simulink model "F16ASYM_Controlled"  (R2015a)
settings: Solver=ode3  SolverMode=SingleTasking  StartTime=0.0  StopTime=inf  FixedStep=T_sim  RelTol=1e-3
InitFcn:
  | load('NN_c_weights_Last_stable.mat')
StopFcn:
  | Final_results
values from neighbouring files (symbols this model uses):
  a1 = fitresult.p1    [Stall_protection.m]
  alpha_map_eval = ones(size(M_eval))*NaN    [Auto_trim_aid.m]    (also in Autotrim_maps.mat = [nan nan 0.277598136245 0.119432432992 0.0579479097061 0.027)
  beta_map_eval = ones(size(M_eval))*NaN    [Auto_trim_aid.m]    (also in Autotrim_maps.mat = [nan nan -0.00151549403324 0.00117807579006 -0.0052086799721)
  C_L_0 = fitresult.p2    [Stall_protection.m]
  G_eval = NaN*ones(size(M_sq,2),size(H_sq,2))    [Stall_protection.m]
  H_sq = unique(sort(H_sq))    [Stall_protection.m]
  H_sq_autotrim = min( F_envelope.H_1g):2000:max(F_envelope.H_1g)    [Auto_trim_aid.m]    (also in Autotrim_maps.mat = [0 2000 4000 6000 8000 10000 12000 14000 16000 18000])
  K_b_q_extrap_ACC = K_b_q_extrap    [RUN_ME.m]
  K_b_q_extrap_AoA = K_b_q_extrap    [RUN_ME.m]
  M_sq = unique(sort(M_sq))    [Stall_protection.m]
  M_sq_autotrim = 0:0.1:max(F_envelope.M_1g)    [Auto_trim_aid.m]    (also in Autotrim_maps.mat = [0 0.1 0.2 0.3 0.4 0.5 0.6 0.7 0.8 0.9 1 1.1 ... (21 element)
  T_sim = 0.02    [RUN_ME.m]
  tau_q_extrap_ACC = tau_q_extrap    [RUN_ME.m]
  tau_q_extrap_AoA = tau_q_extrap    [RUN_ME.m]
  velocity = M_eval(I,J)*a    [Auto_trim_aid.m]
undefined symbols (not defined in the file or in its folder): ACCEL, B, Earth, fi_flag_Simulink, GYRO, H_sq_sche, k_B, K_b_ACC_extrap, K_b_AoA_extrap, latitude, longitude, m, m_B, M_sq_sche, Model_used_flag, rad, s, sigbuilder_block, Stall_curve, tau_ACC_extrap, tau_AoA_extrap, Theta_1_roll_last, Theta_2_roll_last, Theta_3_roll_last, trim_control, trim_state, trim_throttle, V_Comp_A_w_z_last, V_Comp_last, V_Comp_last_ONE, V_long_lastA_w_z, V_long_lastAoA, V_roll_last, V_roll_lastMOD, V_yaw_last, W_Comp_A_w_z_last, W_Comp_last, W_long_lastA_w_z, W_long_lastAoA, W_roll_last, W_roll_lastMOD, W_yaw_last, WGS84
libraries: Adaptive_FaultTolerantControl x57, dspsigops x37, F16_Actuator_Library x14, commnoisgen2 x13, simulink x11, simulink_extras x10, dsparch4 x6, aerolibatmos2 x6, aerolibtransform2 x6, aerolibfltsims x3, dspvision x3, dspsnks4 x3
(part 11 of 14)

== system F16ASYM_Controlled/Primary Controller/P con  + Crossed NN + AWU+Lim + hand-over+Scheduling/P controller + adaptive Crossed NN + AWU+Lim   in AoA/Physical limitation/Moments ==
  C_L : Inport
  C_M : Inport  Port=2
  C_N : Inport  Port=3
  q : Inport  Port=4
  B span : Constant  Value=9.144
  CMA : Constant  Value=3.45
  Divide : Product  Inputs=**
  Divide1 : Product  Inputs=***
  Divide2 : Product  Inputs=**
  Divide3 : Product  Inputs=***
  Divide4 : Product  Inputs=**
  S_w : Constant  Value=27.87
  S_w1 : Constant  Value=27.87
  q1 : InportShadow  Port=4
  L : Outport
  M : Outport  Port=2
  N : Outport  Port=3
  wires:
  q/1 -> Divide1/1
  S_w/1 -> Divide1/2
  B span/1 -> Divide1/3
  C_L/1 -> Divide/1
  Divide1/1 -> Divide2/1, Divide/2
  Divide/1 -> L/1  "L"
  C_N/1 -> Divide2/2
  Divide2/1 -> N/1  "N"
  q1/1 -> Divide3/1
  S_w1/1 -> Divide3/2
  CMA/1 -> Divide3/3
  C_M/1 -> Divide4/1
  Divide3/1 -> Divide4/2
  Divide4/1 -> M/1  "M"

== system F16ASYM_Controlled/Primary Controller/P con + Crossed NN + AWU+Lim + hand-over/P controller + adaptive Crossed NN + AWU+Lim    in ACC /Long Dyn Inversion: alpha_dot ->q/Completed ==
  alpha_dot_c : Inport
  All_meas : Inport  Port=2
  A_w_z : Selector  InputPortWidth=3  Indices=3
  Add : Sum
  Bus Selector : BusSelector  OutputSignals=signal1.AoA meas (rad),signal1.omega_b meas (rad/s),signal1.SS meas (rad),signal1.V_TAS (m/s),signal2.A_w_CG
  Display : Display
  Display1 : Display
  Display2 : Display
  Divide{,1..3} (4 alike) : Product  Inputs=**
  Divide4 : Product  Inputs=/*
  Selector : Selector  InputPortWidth=3
  Selector1 : Selector  InputPortWidth=3  Indices=3
  Trigonometric Function : Trigonometry  Operator=sincos
  Trigonometric Function1 : Trigonometry  Operator=tan
  Trigonometric Function2 : Trigonometry  Operator=cos
  "q_c " : Sum  Inputs=++-
  q_c : Outport
  wires:
  Trigonometric Function/1 -> Divide1/1
  Bus Selector/1 -> Trigonometric Function/1  "<AoA meas (rad)>"
  Selector/1 -> Divide/2
  Bus Selector/2 -> Selector1/1, Selector/1  "<omega_b meas (rad/s)>"
  Divide2/1 -> "q_c "/2, Display1/1
  Selector1/1 -> Divide1/2
  Divide3/1 -> Divide4/1
  alpha_dot_c/1 -> "q_c "/1, Display/1
  All_meas/1 -> Bus Selector/1
  Bus Selector/5 -> A_w_z/1  "<A_w_CG>"
  Bus Selector/3 -> Trigonometric Function1/1, Trigonometric Function2/1  "<SS meas (rad)>"
  Divide4/1 -> "q_c "/3
  "q_c "/1 -> q_c/1
  Divide/1 -> Add/1
  Bus Selector/4 -> Divide3/2  "<V_TAS (m/s)>"
  Add/1 -> Divide2/1
  Trigonometric Function1/1 -> Divide2/2
  Divide1/1 -> Add/2
  Trigonometric Function2/1 -> Divide3/1
  Trigonometric Function/2 -> Divide/1
  A_w_z/1 -> Display2/1, Divide4/2

== system F16ASYM_Controlled/Primary Controller/P con + Crossed NN + AWU+Lim + hand-over/P controller + adaptive Crossed NN + AWU+Lim    in ACC /Long Dyn Inversion: alpha_dot ->q/Simplified ==
  alpha_dot_c : Inport
  All_meas : Inport  Port=2
  A_b_z : Selector  InputPortWidth=3  Indices=3
  Bus Selector : BusSelector  OutputSignals=signal2.A_b_CG,signal1.V_TAS (m/s)
  Display : Display
  Divide4 : Product  Inputs=*/
  "q_c " : Sum  Inputs=+-
  q_c : Outport
  wires:
  "q_c "/1 -> q_c/1
  All_meas/1 -> Bus Selector/1
  alpha_dot_c/1 -> "q_c "/1, Display/1
  Bus Selector/2 -> Divide4/2  "<V_TAS (m/s)>"
  Divide4/1 -> "q_c "/2
  A_b_z/1 -> Divide4/1  "A_b_z"
  Bus Selector/1 -> A_b_z/1  "<A_b_CG>"

== system F16ASYM_Controlled/Primary Controller/P con + Crossed NN + AWU+Lim + hand-over/P controller + adaptive Crossed NN + AWU+Lim    in ACC /Longitudinal controller in A_w_z/Accel rate --> AoA rate! ==
  All_meas : Inport
  1/a_1 : Gain  Gain=1/a1
  Bus Selector : BusSelector  OutputSignals=signal2.q (Pa)
  Divide : Product  Inputs=**
  Divide2 : Product  Inputs=*/
  S : Constant  Value=27.87
  mass : Constant  Value=9295.44
  A_w  to AoA rates factor : Outport
  wires:
  S/1 -> Divide/1
  Bus Selector/1 -> Divide/2  "<q (Pa)>"
  mass/1 -> Divide2/1
  Divide/1 -> Divide2/2
  Divide2/1 -> 1/a_1/1
  All_meas/1 -> Bus Selector/1
  1/a_1/1 -> A_w  to AoA rates factor/1

== system F16ASYM_Controlled/Primary Controller/P con + Crossed NN + AWU+Lim + hand-over/P controller + adaptive Crossed NN + AWU+Lim    in ACC /Longitudinal controller in A_w_z/Stall protection ==
  alpha_dot des : Inport
  All meas : Inport  Port=2
  Bus Selector : BusSelector  OutputSignals=signal1.AoA meas (rad)
  MATLAB Function : MATLAB Function  TreatAsAtomicUnit=on
  AoA des : Outport
  wires:
  alpha_dot des/1 -> MATLAB Function/1(alpha_dot)
  MATLAB Function/1(alpha_dot_out) -> AoA des/1
  All meas/1 -> Bus Selector/1
  Bus Selector/1 -> MATLAB Function/2(alpha)  "<AoA meas (rad)>"

== system F16ASYM_Controlled/Primary Controller/P con + Crossed NN + AWU+Lim + hand-over/P controller + adaptive Crossed NN + AWU+Lim    in ACC /Physical limitation/Moments ==
  C_L : Inport
  C_M : Inport  Port=2
  C_N : Inport  Port=3
  q : Inport  Port=4
  B span : Constant  Value=9.144
  CMA : Constant  Value=3.45
  Divide : Product  Inputs=**
  Divide1 : Product  Inputs=***
  Divide2 : Product  Inputs=**
  Divide3 : Product  Inputs=***
  Divide4 : Product  Inputs=**
  S_w : Constant  Value=27.87
  S_w1 : Constant  Value=27.87
  q1 : InportShadow  Port=4
  L : Outport
  M : Outport  Port=2
  N : Outport  Port=3
  wires:
  Divide4/1 -> M/1  "M"
  Divide3/1 -> Divide4/2
  C_M/1 -> Divide4/1
  CMA/1 -> Divide3/3
  S_w1/1 -> Divide3/2
  q1/1 -> Divide3/1
  Divide2/1 -> N/1  "N"
  C_N/1 -> Divide2/2
  Divide/1 -> L/1  "L"
  Divide1/1 -> Divide/2, Divide2/1
  C_L/1 -> Divide/1
  B span/1 -> Divide1/3
  S_w/1 -> Divide1/2
  q/1 -> Divide1/1

== system F16ASYM_Controlled/Primary Controller/P con + Crossed NN + AWU+Lim + hand-over/P controller + adaptive Crossed NN + AWU+Lim   in AoA/Long Dyn Inversion: alpha_dot ->q/Completed ==
  alpha_dot_c : Inport
  All_meas : Inport  Port=2
  A_w_z : Selector  InputPortWidth=3  Indices=3
  Add : Sum
  Bus Selector : BusSelector  OutputSignals=signal1.AoA meas (rad),signal1.omega_b meas (rad/s),signal1.SS meas (rad),signal1.V_TAS (m/s),signal2.A_w_CG
  Display : Display
  Display1 : Display
  Display2 : Display
  Divide{,1..3} (4 alike) : Product  Inputs=**
  Divide4 : Product  Inputs=/*
  Selector : Selector  InputPortWidth=3
  Selector1 : Selector  InputPortWidth=3  Indices=3
  Trigonometric Function : Trigonometry  Operator=sincos
  Trigonometric Function1 : Trigonometry  Operator=tan
  Trigonometric Function2 : Trigonometry  Operator=cos
  "q_c " : Sum  Inputs=++-
  q_c : Outport
  wires:
  Trigonometric Function/1 -> Divide1/1
  Bus Selector/1 -> Trigonometric Function/1  "<AoA meas (rad)>"
  Selector/1 -> Divide/2
  Bus Selector/2 -> Selector1/1, Selector/1  "<omega_b meas (rad/s)>"
  Divide2/1 -> "q_c "/2, Display1/1
  Selector1/1 -> Divide1/2
  Divide3/1 -> Divide4/1
  alpha_dot_c/1 -> "q_c "/1, Display/1
  All_meas/1 -> Bus Selector/1
  Bus Selector/5 -> A_w_z/1  "<A_w_CG>"
  Bus Selector/3 -> Trigonometric Function1/1, Trigonometric Function2/1  "<SS meas (rad)>"
  Divide4/1 -> "q_c "/3
  "q_c "/1 -> q_c/1
  Divide/1 -> Add/1
  Bus Selector/4 -> Divide3/2  "<V_TAS (m/s)>"
  Add/1 -> Divide2/1
  Trigonometric Function1/1 -> Divide2/2
  Divide1/1 -> Add/2
  Trigonometric Function2/1 -> Divide3/1
  Trigonometric Function/2 -> Divide/1
  A_w_z/1 -> Display2/1, Divide4/2

== system F16ASYM_Controlled/Primary Controller/P con + Crossed NN + AWU+Lim + hand-over/P controller + adaptive Crossed NN + AWU+Lim   in AoA/Long Dyn Inversion: alpha_dot ->q/Simplified ==
  alpha_dot_c : Inport
  All_meas : Inport  Port=2
  A_b_z : Selector  InputPortWidth=3  Indices=3
  Bus Selector : BusSelector  OutputSignals=signal2.A_b_CG,signal1.V_TAS (m/s)
  Display : Display
  Divide4 : Product  Inputs=*/
  "q_c " : Sum  Inputs=+-
  q_c : Outport
  wires:
  "q_c "/1 -> q_c/1
  All_meas/1 -> Bus Selector/1
  alpha_dot_c/1 -> "q_c "/1, Display/1
  Bus Selector/2 -> Divide4/2  "<V_TAS (m/s)>"
  Divide4/1 -> "q_c "/2
  A_b_z/1 -> Divide4/1  "A_b_z"
  Bus Selector/1 -> A_b_z/1  "<A_b_CG>"

== system F16ASYM_Controlled/Primary Controller/P con + Crossed NN + AWU+Lim + hand-over/P controller + adaptive Crossed NN + AWU+Lim   in AoA/Physical limitation/Moments ==
  C_L : Inport
  C_M : Inport  Port=2
  C_N : Inport  Port=3
  q : Inport  Port=4
  B span : Constant  Value=9.144
  CMA : Constant  Value=3.45
  Divide : Product  Inputs=**
  Divide1 : Product  Inputs=***
  Divide2 : Product  Inputs=**
  Divide3 : Product  Inputs=***
  Divide4 : Product  Inputs=**
  S_w : Constant  Value=27.87
  S_w1 : Constant  Value=27.87
  q1 : InportShadow  Port=4
  L : Outport
  M : Outport  Port=2
  N : Outport  Port=3
  wires:
  Divide4/1 -> M/1  "M"
  Divide3/1 -> Divide4/2
  C_M/1 -> Divide4/1
  CMA/1 -> Divide3/3
  S_w1/1 -> Divide3/2
  q1/1 -> Divide3/1
  Divide2/1 -> N/1  "N"
  C_N/1 -> Divide2/2
  Divide/1 -> L/1  "L"
  Divide1/1 -> Divide/2, Divide2/1
  C_L/1 -> Divide/1
  B span/1 -> Divide1/3
  S_w/1 -> Divide1/2
  q/1 -> Divide1/1

== system F16ASYM_Controlled/Primary Controller/P con + adaptive Crossed NN + AWU+Lim + Scheduling/Body Rates Controller/Body Rates Controller  in ACC/Ref Model and P Controller1 ==
  y_ref : Inport
  y_meas : Inport  Port=2
  All meas : Inport  Port=3
  " " : Sum  Inputs=|+-
  2-D Lookup Table1 : Lookup_n-D  BreakpointsForDimension1=M_sq_sche  BreakpointsForDimension2=H_sq_sche  BeginIndexSearchUsingPreviousIndexResult=on  Table=tau_q_extrap_ACC  ExtrapMethod=Clip  RemoveProtectionInput=on  UseLastTableValue=on  SampleTime=2*T_sim  RndMeth=Simplest  InputSameDT=on
  2-D Lookup Table2 : Lookup_n-D  BreakpointsForDimension1=M_sq_sche  BreakpointsForDimension2=H_sq_sche  BeginIndexSearchUsingPreviousIndexResult=on  Table=K_b_q_extrap_ACC  ExtrapMethod=Clip  RemoveProtectionInput=on  UseLastTableValue=on  SampleTime=2*T_sim  RndMeth=Simplest  InputSameDT=on
  Add1 : Sum  Inputs=++|
  Bus Selector1 : BusSelector  OutputSignals=signal2.Mach,signal1.Alt meas (m)
  Divide : Product  Inputs=**
  K_f : Gain
  Reference Model : Subsystem
  Saturation : Saturate  UpperLimit=1  LowerLimit=2*T_sim
  Saturation1 : Saturate  UpperLimit=10  LowerLimit=0.1
  Switch1 : Switch  Threshold=0.5
  Switch2 : Switch  Threshold=0.5
  def : Constant
  isNaN1 : RelationalOperator  Operator=isNaN  OutDataTypeStr=boolean
  isNaN2 : RelationalOperator  Operator=isNaN  OutDataTypeStr=boolean
  max : Constant  Value=0.6
  y_des_dot : Outport
  y_c_ff_dot : Outport  Port=2
  y_c : Outport  Port=3
  y_meas_out : Outport  Port=4
  k_b param : Outport  Port=5
  wires:
  Saturation1/1 -> k_b param/1, Divide/2
  y_meas/1 -> y_meas_out/1, " "/2
  Reference Model/2(y_c) -> y_c/1, " "/1
  " "/1 -> Divide/1
  y_ref/1 -> Reference Model/1(y_ref)
  Add1/1 -> y_des_dot/1
  Reference Model/1(y_c_dot) -> K_f/1
  K_f/1 -> y_c_ff_dot/1, Add1/1
  Divide/1 -> Add1/2
  All meas/1 -> Bus Selector1/1
  Bus Selector1/1 -> 2-D Lookup Table2/1, 2-D Lookup Table1/1  "<Mach>"
  Bus Selector1/2 -> 2-D Lookup Table2/2, 2-D Lookup Table1/2  "<Alt meas (m)>"
  max/1 -> Switch1/1
  isNaN2/1 -> Switch1/2
  2-D Lookup Table1/1 -> Switch1/3, isNaN2/1
  Switch1/1 -> Saturation/1
  def/1 -> Switch2/1
  isNaN1/1 -> Switch2/2
  2-D Lookup Table2/1 -> isNaN1/1, Switch2/3
  Saturation/1 -> Reference Model/2(tau)
  Switch2/1 -> Saturation1/1

== system F16ASYM_Controlled/Primary Controller/P con + adaptive Crossed NN + AWU+Lim + Scheduling/Body Rates Controller/Body Rates Controller in  AoA/Ref Model and P Controller1 ==
  y_ref : Inport
  y_meas : Inport  Port=2
  All meas : Inport  Port=3
  " " : Sum  Inputs=|+-
  2-D Lookup Table1 : Lookup_n-D  BreakpointsForDimension1=M_sq_sche  BreakpointsForDimension2=H_sq_sche  BeginIndexSearchUsingPreviousIndexResult=on  Table=tau_q_extrap_AoA  ExtrapMethod=Clip  RemoveProtectionInput=on  UseLastTableValue=on  SampleTime=2*T_sim  RndMeth=Simplest  InputSameDT=on
  2-D Lookup Table2 : Lookup_n-D  BreakpointsForDimension1=M_sq_sche  BreakpointsForDimension2=H_sq_sche  BeginIndexSearchUsingPreviousIndexResult=on  Table=K_b_q_extrap_AoA  ExtrapMethod=Clip  RemoveProtectionInput=on  UseLastTableValue=on  SampleTime=2*T_sim  RndMeth=Simplest  InputSameDT=on
  Add1 : Sum  Inputs=++|
  Bus Selector1 : BusSelector  OutputSignals=signal2.Mach,signal1.Alt meas (m)
  Divide : Product  Inputs=**
  K_f : Gain
  Reference Model : Subsystem
  Saturation : Saturate  UpperLimit=0.14  LowerLimit=2*T_sim
  Saturation1 : Saturate  UpperLimit=4  LowerLimit=0.1
  Switch1 : Switch  Threshold=0.5
  Switch2 : Switch  Threshold=0.5
  def : Constant  Value=2.83
  isNaN1 : RelationalOperator  Operator=isNaN  OutDataTypeStr=boolean
  isNaN2 : RelationalOperator  Operator=isNaN  OutDataTypeStr=boolean
  max : Constant  Value=0.1
  y_des_dot : Outport
  y_c_ff_dot : Outport  Port=2
  y_c : Outport  Port=3
  y_meas_out : Outport  Port=4
  k_b param : Outport  Port=5
  wires:
  Saturation1/1 -> k_b param/1, Divide/2
  y_meas/1 -> y_meas_out/1, " "/2
  Reference Model/2(y_c) -> y_c/1, " "/1
  " "/1 -> Divide/1
  y_ref/1 -> Reference Model/1(y_ref)
  Add1/1 -> y_des_dot/1
  Reference Model/1(y_c_dot) -> K_f/1
  K_f/1 -> y_c_ff_dot/1, Add1/1
  Divide/1 -> Add1/2
  All meas/1 -> Bus Selector1/1
  Bus Selector1/1 -> 2-D Lookup Table2/1, 2-D Lookup Table1/1  "<Mach>"
  Bus Selector1/2 -> 2-D Lookup Table2/2, 2-D Lookup Table1/2  "<Alt meas (m)>"
  max/1 -> Switch1/1
  isNaN2/1 -> Switch1/2
  2-D Lookup Table1/1 -> Switch1/3, isNaN2/1
  Switch1/1 -> Saturation/1
  def/1 -> Switch2/1
  isNaN1/1 -> Switch2/2
  2-D Lookup Table2/1 -> isNaN1/1, Switch2/3
  Saturation/1 -> Reference Model/2(tau)
  Switch2/1 -> Saturation1/1

== system F16ASYM_Controlled/Primary Controller/P con + adaptive Crossed NN + AWU+Lim + Scheduling/Longitudinal Controller: AoA or A_w_z/Longitudinal controller in A_w_z/Accel rate --> AoA rate! ==
  All_meas : Inport
  1/a_1 : Gain  Gain=1/a1
  Bus Selector : BusSelector  OutputSignals=signal2.q (Pa)
  Divide : Product  Inputs=**
  Divide2 : Product  Inputs=*/
  S : Constant  Value=27.87
  mass : Constant  Value=9295.44
  A_w  to AoA rates factor : Outport
  wires:
  1/a_1/1 -> A_w  to AoA rates factor/1
  All_meas/1 -> Bus Selector/1
  Divide2/1 -> 1/a_1/1
  Divide/1 -> Divide2/2
  mass/1 -> Divide2/1
  Bus Selector/1 -> Divide/2  "<q (Pa)>"
  S/1 -> Divide/1

== system F16ASYM_Controlled/Primary Controller/P con + adaptive Crossed NN + AWU+Lim + Scheduling/Longitudinal Controller: AoA or A_w_z/Longitudinal controller in A_w_z/Ref Model and P Controller1 ==
  y_ref : Inport
  y_meas : Inport  Port=2
  All meas : Inport  Port=3
  " " : Sum  Inputs=|+-
  2-D Lookup Table1 : Lookup_n-D  BreakpointsForDimension1=M_sq_sche  BreakpointsForDimension2=H_sq_sche  BeginIndexSearchUsingPreviousIndexResult=on  Table=tau_ACC_extrap  ExtrapMethod=Clip  RemoveProtectionInput=on  UseLastTableValue=on  SampleTime=2*T_sim  RndMeth=Simplest  InputSameDT=on
  2-D Lookup Table2 : Lookup_n-D  BreakpointsForDimension1=M_sq_sche  BreakpointsForDimension2=H_sq_sche  BeginIndexSearchUsingPreviousIndexResult=on  Table=K_b_ACC_extrap  ExtrapMethod=Clip  RemoveProtectionInput=on  UseLastTableValue=on  SampleTime=2*T_sim  RndMeth=Simplest  InputSameDT=on
  Add1 : Sum  Inputs=++|
  Bus Selector1 : BusSelector  OutputSignals=signal2.Mach,signal1.Alt meas (m)
  Divide : Product  Inputs=**
  K_f : Gain
  Reference Model : Subsystem
  Saturation : Saturate  UpperLimit=2  LowerLimit=0.1
  Saturation1 : Saturate  UpperLimit=15  LowerLimit=0.1
  Switch1 : Switch  Threshold=0.5
  Switch2 : Switch  Threshold=0.5
  def : Constant
  isNaN1 : RelationalOperator  Operator=isNaN  OutDataTypeStr=boolean
  isNaN2 : RelationalOperator  Operator=isNaN  OutDataTypeStr=boolean
  max : Constant  Value=2.2
  y_des_dot : Outport
  y_c_ff_dot : Outport  Port=2
  y_c : Outport  Port=3
  y_meas_out : Outport  Port=4
  k_b param : Outport  Port=5
  wires:
  Saturation1/1 -> k_b param/1, Divide/2
  y_meas/1 -> y_meas_out/1, " "/2
  Reference Model/2(y_c) -> y_c/1, " "/1
  " "/1 -> Divide/1
  y_ref/1 -> Reference Model/1(y_ref)
  Add1/1 -> y_des_dot/1
  Reference Model/1(y_c_dot) -> K_f/1
  K_f/1 -> y_c_ff_dot/1, Add1/1
  Divide/1 -> Add1/2
  All meas/1 -> Bus Selector1/1
  Bus Selector1/1 -> 2-D Lookup Table2/1, 2-D Lookup Table1/1  "<Mach>"
  Bus Selector1/2 -> 2-D Lookup Table2/2, 2-D Lookup Table1/2  "<Alt meas (m)>"
  max/1 -> Switch1/1
  isNaN2/1 -> Switch1/2
  2-D Lookup Table1/1 -> Switch1/3, isNaN2/1
  Switch1/1 -> Saturation/1
  def/1 -> Switch2/1
  isNaN1/1 -> Switch2/2
  2-D Lookup Table2/1 -> isNaN1/1, Switch2/3
  Saturation/1 -> Reference Model/2(tau)
  Switch2/1 -> Saturation1/1

== system F16ASYM_Controlled/Primary Controller/P con + adaptive Crossed NN + AWU+Lim + Scheduling/Longitudinal Controller: AoA or A_w_z/Longitudinal controller in A_w_z/Stall protection ==
  alpha_dot des : Inport
  All meas : Inport  Port=2
  Bus Selector : BusSelector  OutputSignals=signal1.AoA meas (rad)
  MATLAB Function : MATLAB Function  TreatAsAtomicUnit=on
  AoA des : Outport
  wires:
  Bus Selector/1 -> MATLAB Function/2(alpha)  "<AoA meas (rad)>"
  All meas/1 -> Bus Selector/1
  MATLAB Function/1(alpha_dot_out) -> AoA des/1
  alpha_dot des/1 -> MATLAB Function/1(alpha_dot)

== system F16ASYM_Controlled/Primary Controller/P con + adaptive Crossed NN + AWU+Lim + Scheduling/Longitudinal Controller: AoA or A_w_z/Longitudinal controller in AoA/Ref Model and P Controller1 ==
  y_ref : Inport
  y_meas : Inport  Port=2
  All meas : Inport  Port=3
  " " : Sum  Inputs=|+-
  2-D Lookup Table1 : Lookup_n-D  BreakpointsForDimension1=M_sq_sche  BreakpointsForDimension2=H_sq_sche  BeginIndexSearchUsingPreviousIndexResult=on  Table=tau_AoA_extrap  ExtrapMethod=Clip  RemoveProtectionInput=on  UseLastTableValue=on  SampleTime=2*T_sim  RndMeth=Simplest  InputSameDT=on
  2-D Lookup Table2 : Lookup_n-D  BreakpointsForDimension1=M_sq_sche  BreakpointsForDimension2=H_sq_sche  BeginIndexSearchUsingPreviousIndexResult=on  Table=K_b_AoA_extrap  ExtrapMethod=Clip  RemoveProtectionInput=on  UseLastTableValue=on  SampleTime=2*T_sim  RndMeth=Simplest  InputSameDT=on
  Add1 : Sum  Inputs=++|
  Bus Selector1 : BusSelector  OutputSignals=signal2.Mach,signal1.Alt meas (m)
  Divide : Product  Inputs=**
  K_f : Gain
  Reference Model : Subsystem
  Saturation : Saturate  UpperLimit=1  LowerLimit=0.1
  Saturation1 : Saturate  UpperLimit=15  LowerLimit=0.1
  Switch1 : Switch  Threshold=0.5
  Switch2 : Switch  Threshold=0.5
  def : Constant  Value=5.3
  isNaN1 : RelationalOperator  Operator=isNaN  OutDataTypeStr=boolean
  isNaN2 : RelationalOperator  Operator=isNaN  OutDataTypeStr=boolean
  max : Constant  Value=0.7
  y_des_dot : Outport
  y_c_ff_dot : Outport  Port=2
  y_c : Outport  Port=3
  y_meas_out : Outport  Port=4
  k_b param : Outport  Port=5
  wires:
  Saturation1/1 -> k_b param/1, Divide/2
  y_meas/1 -> y_meas_out/1, " "/2
  Reference Model/2(y_c) -> y_c/1, " "/1
  " "/1 -> Divide/1
  y_ref/1 -> Reference Model/1(y_ref)
  Add1/1 -> y_des_dot/1
  Reference Model/1(y_c_dot) -> K_f/1
  K_f/1 -> y_c_ff_dot/1, Add1/1
  Divide/1 -> Add1/2
  All meas/1 -> Bus Selector1/1
  Bus Selector1/1 -> 2-D Lookup Table2/1, 2-D Lookup Table1/1  "<Mach>"
  Bus Selector1/2 -> 2-D Lookup Table2/2, 2-D Lookup Table1/2  "<Alt meas (m)>"
  max/1 -> Switch1/1
  isNaN2/1 -> Switch1/2
  2-D Lookup Table1/1 -> Switch1/3, isNaN2/1
  Switch1/1 -> Saturation/1
  def/1 -> Switch2/1
  isNaN1/1 -> Switch2/2
  2-D Lookup Table2/1 -> isNaN1/1, Switch2/3
  Saturation/1 -> Reference Model/2(tau)
  Switch2/1 -> Saturation1/1

== system F16ASYM_Controlled/Primary Controller/P cont + adaptive Crossed NN + AWU+Lim /Longitudinal Controller: AoA or A_w_z/Longitudinal controller in A_w_z/Accel rate --> AoA rate! ==
  All_meas : Inport
  1/a_1 : Gain  Gain=1/a1
  Bus Selector : BusSelector  OutputSignals=signal2.q (Pa)
  Divide : Product  Inputs=**
  Divide2 : Product  Inputs=*/
  S : Constant  Value=27.87
  mass : Constant  Value=9295.44
  A_w  to AoA rates factor : Outport
  wires:
  S/1 -> Divide/1
  Bus Selector/1 -> Divide/2  "<q (Pa)>"
  mass/1 -> Divide2/1
  Divide/1 -> Divide2/2
  Divide2/1 -> 1/a_1/1
  All_meas/1 -> Bus Selector/1
  1/a_1/1 -> A_w  to AoA rates factor/1

== system F16ASYM_Controlled/Primary Controller/P cont + adaptive Crossed NN + AWU+Lim /Longitudinal Controller: AoA or A_w_z/Longitudinal controller in A_w_z/Stall protection ==
  alpha_dot des : Inport
  All meas : Inport  Port=2
  Bus Selector : BusSelector  OutputSignals=signal1.AoA meas (rad)
  MATLAB Function : MATLAB Function  TreatAsAtomicUnit=on
  AoA des : Outport
  wires:
  alpha_dot des/1 -> MATLAB Function/1(alpha_dot)
  MATLAB Function/1(alpha_dot_out) -> AoA des/1
  All meas/1 -> Bus Selector/1
  Bus Selector/1 -> MATLAB Function/2(alpha)  "<AoA meas (rad)>"

== system F16ASYM_Controlled/Primary Controller/P cont + adaptive Crossed NN + AWU+Lim ONELAYER/Longitudinal Controller: AoA or A_w_z/Longitudinal controller in A_w_z/Accel rate --> AoA rate! ==
  All_meas : Inport
  1/a_1 : Gain  Gain=1/a1
  Bus Selector : BusSelector  OutputSignals=signal2.q (Pa)
  Divide : Product  Inputs=**
  Divide2 : Product  Inputs=*/
  S : Constant  Value=27.87
  mass : Constant  Value=9295.44
  A_w  to AoA rates factor : Outport
  wires:
  S/1 -> Divide/1
  Bus Selector/1 -> Divide/2  "<q (Pa)>"
  mass/1 -> Divide2/1
  Divide/1 -> Divide2/2
  Divide2/1 -> 1/a_1/1
  All_meas/1 -> Bus Selector/1
  1/a_1/1 -> A_w  to AoA rates factor/1

== system F16ASYM_Controlled/Primary Controller/P cont + adaptive Crossed NN + AWU+Lim ONELAYER/Longitudinal Controller: AoA or A_w_z/Longitudinal controller in A_w_z/Stall protection ==
  alpha_dot des : Inport
  All meas : Inport  Port=2
  Bus Selector : BusSelector  OutputSignals=signal1.AoA meas (rad)
  MATLAB Function : MATLAB Function  TreatAsAtomicUnit=on
  AoA des : Outport
  wires:
  alpha_dot des/1 -> MATLAB Function/1(alpha_dot)
  MATLAB Function/1(alpha_dot_out) -> AoA des/1
  All meas/1 -> Bus Selector/1
  Bus Selector/1 -> MATLAB Function/2(alpha)  "<AoA meas (rad)>"

== system F16ASYM_Controlled/Primary Controller/P controller/Longitudinal Controller: AoA or A_w_z/Longitudinal controller in A_w_z/Accel rate --> AoA rate! ==
  A_w_z dot : Inport
  All_meas : Inport  Port=2
  1/a_1 : Gain  Gain=1/a1
  Bus Selector : BusSelector  OutputSignals=signal2.q (Pa)
  Divide : Product  Inputs=**
  Divide1 : Product  Inputs=**
  Divide2 : Product  Inputs=*/
  S : Constant  Value=27.87
  mass : Constant  Value=9295.44
  alpha_dot des : Outport
  wires:
  1/a_1/1 -> alpha_dot des/1  "ALPHA_DOT"
  All_meas/1 -> Bus Selector/1
  Divide2/1 -> 1/a_1/1
  Divide/1 -> Divide2/2
  Divide1/1 -> Divide2/1
  mass/1 -> Divide1/2
  Bus Selector/1 -> Divide/2  "<q (Pa)>"
  S/1 -> Divide/1
  A_w_z dot/1 -> Divide1/1

== system F16ASYM_Controlled/Primary Controller/P controller + adaptive Crossed NN/Longitudinal Controller: AoA or A_w_z/Longitudinal controller in A_w_z/Accel rate --> AoA rate! ==
  All_meas : Inport
  1/a_1 : Gain  Gain=1/a1
  Bus Selector : BusSelector  OutputSignals=signal2.q (Pa)
  Divide : Product  Inputs=**
  Divide2 : Product  Inputs=*/
  S : Constant  Value=27.87
  mass : Constant  Value=9295.44
  A_w  to AoA rates factor : Outport
  wires:
  1/a_1/1 -> A_w  to AoA rates factor/1
  All_meas/1 -> Bus Selector/1
  Divide2/1 -> 1/a_1/1
  Divide/1 -> Divide2/2
  mass/1 -> Divide2/1
  Bus Selector/1 -> Divide/2  "<q (Pa)>"
  S/1 -> Divide/1

== system F16ASYM_Controlled/Primary Controller/P controller + adaptive Isolated NN/Longitudinal Controller: AoA or A_w_z/Longitudinal controller in A_w_z/Accel rate --> AoA rate! ==
  All_meas : Inport
  1/a_1 : Gain  Gain=1/a1
  Bus Selector : BusSelector  OutputSignals=signal2.q (Pa)
  Divide : Product  Inputs=**
  Divide2 : Product  Inputs=*/
  S : Constant  Value=27.87
  mass : Constant  Value=9295.44
  A_w  to AoA rates factor : Outport
  wires:
  S/1 -> Divide/1
  Bus Selector/1 -> Divide/2  "<q (Pa)>"
  mass/1 -> Divide2/1
  Divide/1 -> Divide2/2
  Divide2/1 -> 1/a_1/1
  All_meas/1 -> Bus Selector/1
  1/a_1/1 -> A_w  to AoA rates factor/1

== system F16ASYM_Controlled/Primary Controller/P controller + adaptive Isolated NN/On-line (adaptive) multi-layer NNs/Long Chanel/Long HL NN A_w_z ==
  note: Be careful with dimensions of inputs!!!
      | NORMALIZATION!!!
  v_ad^ prev : Inport
  Long_chanel vars : Inport  Port=2
  All_meas : Inport  Port=3
  Long_learning rate : Inport  Port=4
  Long reg param : Inport  Port=5
  Bus Selector1 : BusSelector  OutputSignals=A_chanel vars.A_err,q_chanel_vars.q_err,A_chanel vars.A_sf,A_chanel vars.A_sf_dot,q_chanel_vars.q_sf_dot,A_chanel vars.K_b_A,q_chanel_vars.K_b_q,A_chanel vars.FactorF
  Bus Selector2 : BusSelector  OutputSignals=signal1.Alt meas (m),signal2.Mach
  Constant : Constant
  Constant1 : Constant  Value=[0;1]
  Divide : Product  Inputs=**
  Long NN : MATLAB Function  TreatAsAtomicUnit=on
  Memory2 : Memory  X0=V_long_lastA_w_z
  Memory3 : Memory  X0=W_long_lastA_w_z
  Mux : Mux  Inputs=10
  Mux1 : Mux  Inputs=2
  Mux2 : Mux  Inputs=2
  Scope : Scope
      settings: YMin=0  YMax=0.003  SaveName=ScopeData13
  Terminator : Terminator
  Terminator1 : Terminator
  To Workspace : ToWorkspace  VariableName=V_long_lastA_w_z  SampleTime=-1
      settings: MaxDataPoints=1
  To Workspace1 : ToWorkspace  VariableName=W_long_lastA_w_z  SampleTime=-1
      settings: MaxDataPoints=1
  dim-less : Gain  Gain=T_sim
  dim-less1 : Gain  Gain=T_sim^2
  scaling : Gain  Gain=1/15000
  scaling1 : Gain  Gain=1/(9*9.81)
  scaling2 : Gain  Gain=1/(9*9.81)
  scaling3 : Gain  Gain=1/(9*9.81)
  v_ad_comp : Outport
  wires:
  Long NN/2(v_ad) -> Terminator/1
  Long NN/5(V_update) -> To Workspace/1, Memory2/1
  v_ad^ prev/1 -> Mux/10
  [Ks] -> Long NN/4(Ks)
  Constant1/1 -> Long NN/5(B)
  Memory3/1 -> Long NN/8(W)
  Memory2/1 -> Long NN/9(V)
  Long NN/4(W_update) -> To Workspace1/1, Memory3/1
  Long NN/1(v_ad_comp) -> v_ad_comp/1
  Mux/1 -> Scope/1, Long NN/1(X_bar)
  Long_chanel vars/1 -> Bus Selector1/1
  Long_learning rate/1 -> Long NN/6(Long_learnign_rate)
  Long reg param/1 -> Long NN/7(Long_reg_param)
  Constant/1 -> Mux/1
  All_meas/1 -> Bus Selector2/1
  Bus Selector2/1 -> scaling/1  "<Alt meas (m)>"
  Divide/1 -> Mux/4
  scaling/1 -> Mux/2
  Bus Selector2/2 -> Mux/3, Divide/2, Divide/1  "<Mach>"
  Bus Selector1/1 -> Mux1/1, scaling2/1  "<A_err>"
  Bus Selector1/2 -> Mux1/2, Mux/6  "<q_err>"
  Bus Selector1/3 -> scaling1/1  "<A_sf>"
  Bus Selector1/4 -> dim-less/1  "<A_sf_dot>"
  Bus Selector1/5 -> dim-less1/1  "<q_sf_dot>"
  Mux1/1 -> Long NN/2(e)  "e"
  Bus Selector1/7 -> Mux2/2  "<K_b_q>"
  Bus Selector1/6 -> Mux2/1  "<K_b_A>"
  Mux2/1 -> [Ks]
  Bus Selector1/8 -> Long NN/3(F)  "<FactorF>"
  scaling2/1 -> Mux/5
  scaling1/1 -> Mux/7
  scaling3/1 -> Mux/8
  Long NN/3(Z_norm_unit) -> Terminator1/1
  dim-less/1 -> scaling3/1
  dim-less1/1 -> Mux/9

== system F16ASYM_Controlled/Primary Controller/P controller + adaptive Isolated NN/On-line (adaptive) multi-layer NNs/Long Chanel/Long HL NN AoA ==
  note: Be careful with dimensions of inputs!!!
      | NORMALIZATION!!!
  v_ad^ prev : Inport
  Long_chanel vars : Inport  Port=2
  All_meas : Inport  Port=3
  Long_learning rate : Inport  Port=4
  Long reg param : Inport  Port=5
  Bus Selector1 : BusSelector  OutputSignals=alpha_chanel vars.alpha_err,q_chanel_vars.q_err,alpha_chanel vars.alpha_sf,alpha_chanel vars.alpha_sf_dot,q_chanel_vars.q_sf_dot,alpha_chanel vars.K_b_alpha,q_chanel_vars.K_b_q
  Bus Selector2 : BusSelector  OutputSignals=signal1.Alt meas (m),signal2.Mach
  Constant : Constant
  Constant1 : Constant  Value=[0;1]
  Display : Display
  Divide : Product  Inputs=**
  Gain : Gain  Gain=1/15000
  Long NN : MATLAB Function  TreatAsAtomicUnit=on
  Memory2 : Memory  X0=V_long_lastAoA
  Memory3 : Memory  X0=W_long_lastAoA
  Mux : Mux  Inputs=10
  Mux1 : Mux  Inputs=2
  Mux2 : Mux  Inputs=2
  Scope : Scope
      settings: YMin=-0.7  YMax=1  SaveName=ScopeData18
  Terminator : Terminator
  Terminator1 : Terminator
  To Workspace : ToWorkspace  VariableName=V_long_lastAoA  SampleTime=-1
      settings: MaxDataPoints=1
  To Workspace1 : ToWorkspace  VariableName=W_long_lastAoA  SampleTime=-1
      settings: MaxDataPoints=1
  dem-less : Gain  Gain=T_sim
  dem-less1 : Gain  Gain=T_sim^2
  v_ad_comp : Outport
  wires:
  Long NN/2(v_ad) -> Terminator/1
  Long NN/5(V_update) -> To Workspace/1, Memory2/1
  v_ad^ prev/1 -> Mux/10
  [Ks] -> Long NN/3(Ks)
  Constant1/1 -> Long NN/4(B)
  Memory3/1 -> Long NN/7(W)
  Memory2/1 -> Long NN/8(V)
  Long NN/4(W_update) -> To Workspace1/1, Memory3/1
  Long NN/1(v_ad_comp) -> v_ad_comp/1
  Long_chanel vars/1 -> Bus Selector1/1
  Long_learning rate/1 -> Long NN/5(Long_learnign_rate)
  Long reg param/1 -> Long NN/6(Long_reg_param)
  Constant/1 -> Mux/1
  All_meas/1 -> Bus Selector2/1
  Bus Selector2/1 -> Gain/1  "<Alt meas (m)>"
  Divide/1 -> Mux/4
  Gain/1 -> Mux/2
  Bus Selector2/2 -> Mux/3, Divide/2, Divide/1  "<Mach>"
  Bus Selector1/1 -> Mux1/1, Mux/5  "<alpha_err>"
  Bus Selector1/2 -> Mux1/2, Mux/6  "<q_err>"
  Bus Selector1/3 -> Mux/7  "<alpha_sf>"
  Bus Selector1/4 -> dem-less/1  "<alpha_sf_dot>"
  Bus Selector1/5 -> dem-less1/1  "<q_sf_dot>"
  Mux1/1 -> Long NN/2(e)  "e"
  Bus Selector1/7 -> Mux2/2  "<K_b_q>"
  Bus Selector1/6 -> Mux2/1  "<K_b_alpha>"
  Mux2/1 -> [Ks]
  Long NN/3(Z_norm_unit) -> Terminator1/1
  Mux/1 -> Scope/1, Display/1, Long NN/1(X_bar)
  dem-less/1 -> Mux/8
  dem-less1/1 -> Mux/9

== system F16ASYM_Controlled/Primary Controller/P controller + adaptive Isolated NN/On-line (adaptive) multi-layer NNs/Roll NN/Roll 1HL NN ==
  note: Be careful with dimensions of inputs!!!
      | NORMALIZATION!!!
  v_ad^ prev : Inport
  p_chanel vars : Inport  Port=2
  All_meas : Inport  Port=3
  Roll_learning rate : Inport  Port=4
  Roll reg param : Inport  Port=5
  Bus Selector1 : BusSelector  OutputSignals=p_err,p_sf,p_sf_dot,K_b_p
  Bus Selector2 : BusSelector  OutputSignals=signal1.Alt meas (m),signal2.Mach,signal1.AoA meas (rad),signal1.SS meas (rad),signal1.omega_b meas (rad/s)
  Constant : Constant
  Constant1 : Constant
  Constant2 : Constant
  Display : Display
  Divide : Product  Inputs=**
  Divide1 : Product  Inputs=**
  Divide2 : Product  Inputs=*/
  Memory2 : Memory  X0=V_roll_last
  Memory3 : Memory  X0=W_roll_last
  Mux : Mux  Inputs=12
  Roll NN : MATLAB Function  TreatAsAtomicUnit=on
  Scope : Scope
      settings: YMin=-0.5  YMax=6  SaveName=ScopeData15
  Selector : Selector  InputPortWidth=3  Indices=3
  Terminator : Terminator
  Terminator1 : Terminator
  To Workspace : ToWorkspace  VariableName=V_roll_last  SampleTime=-1
      settings: MaxDataPoints=1
  To Workspace1 : ToWorkspace  VariableName=W_roll_last  SampleTime=-1
      settings: MaxDataPoints=1
  dem-less : Gain  Gain=T_sim
  dim-less : Gain  Gain=1/15000
  v_ad_comp : Outport
  wires:
  Constant2/1 -> Divide2/1
  Bus Selector1/4 -> Divide2/2  "<K_b_p>"
  Divide2/1 -> [P]
  Roll NN/2(v_ad) -> Terminator/1
  Roll NN/5(V_update) -> To Workspace/1, Memory2/1
  v_ad^ prev/1 -> Mux/12
  [P] -> Roll NN/3(P)
  Constant1/1 -> Roll NN/4(B)
  Memory3/1 -> Roll NN/7(W)
  Memory2/1 -> Roll NN/8(V)
  Roll NN/4(W_update) -> To Workspace1/1, Memory3/1
  Roll NN/1(v_ad_comp) -> v_ad_comp/1
  Mux/1 -> Roll NN/1(X_bar), Scope/1, Display/1
  Bus Selector1/1 -> Mux/9, Roll NN/2(e)  "<p_err>"
  Bus Selector1/3 -> dem-less/1  "<p_sf_dot>"
  Bus Selector1/2 -> Mux/10  "<p_sf>"
  p_chanel vars/1 -> Bus Selector1/1
  Roll_learning rate/1 -> Roll NN/5(Roll_learnign_rate)
  Roll reg param/1 -> Roll NN/6(Roll_reg_param)
  Constant/1 -> Mux/1
  All_meas/1 -> Bus Selector2/1
  Bus Selector2/1 -> dim-less/1  "<Alt meas (m)>"
  Divide/1 -> Mux/4
  Bus Selector2/3 -> Divide1/2, Divide1/1, Mux/5  "<AoA meas (rad)>"
  Divide1/1 -> Mux/6
  Bus Selector2/4 -> Mux/7  "<SS meas (rad)>"
  dim-less/1 -> Mux/2
  Bus Selector2/5 -> Selector/1  "<omega_b meas (rad/s)>"
  Selector/1 -> Mux/8
  Bus Selector2/2 -> Divide/2, Divide/1, Mux/3  "<Mach>"
  Roll NN/3(Z_norm_unit) -> Terminator1/1
  dem-less/1 -> Mux/11

== system F16ASYM_Controlled/Primary Controller/P controller + adaptive Isolated NN/On-line (adaptive) multi-layer NNs/Roll NN/Roll 2HL NN ==
  note: Be careful with dimensions of inputs!!!
      | NORMALIZATION!!!
  v_ad^ prev : Inport
  p_chanel vars : Inport  Port=2
  All_meas : Inport  Port=3
  Roll_learning rate : Inport  Port=4
  Roll reg param : Inport  Port=5
  " " : ToWorkspace  VariableName=Theta_3_roll_last  SampleTime=-1
      settings: MaxDataPoints=1
  "  " : Memory  X0=Theta_3_roll_last
  "   " : Memory  X0=Theta_2_roll_last
  B : Constant
  Bus Selector1 : BusSelector  OutputSignals=p_err,p_sf,p_sf_dot,K_b_p
  Bus Selector2 : BusSelector  OutputSignals=signal1.Alt meas (m),signal2.Mach,signal1.AoA meas (rad),signal1.SS meas (rad),signal1.omega_b meas (rad/s)
  Constant : Constant
  Constant2 : Constant
  Display : Display
  Divide : Product  Inputs=**
  Divide1 : Product  Inputs=**
  Divide2 : Product  Inputs=*/
  Gain : Gain  Gain=1/15000
  Memory2 : Memory  X0=Theta_1_roll_last
  Mux : Mux  Inputs=12
  Roll Multilayer NN : MATLAB Function  TreatAsAtomicUnit=on
  Scope : Scope
      settings: YMin=-14  YMax=4  SaveName=ScopeData16
  Selector : Selector  InputPortWidth=3  Indices=3
  Terminator : Terminator
  Terminator1 : Terminator
  To Workspace : ToWorkspace  VariableName=Theta_1_roll_last  SampleTime=-1
      settings: MaxDataPoints=1
  To Workspace1 : ToWorkspace  VariableName=Theta_2_roll_last  SampleTime=-1
      settings: MaxDataPoints=1
  dem-less : Gain  Gain=T_sim
  v_ad_comp : Outport
  wires:
  p_chanel vars/1 -> Bus Selector1/1
  Bus Selector1/2 -> Mux/10  "<p_sf>"
  Bus Selector1/3 -> dem-less/1  "<p_sf_dot>"
  Bus Selector1/1 -> Mux/9, Roll Multilayer NN/2(e)  "<p_err>"
  Constant/1 -> Mux/1
  All_meas/1 -> Bus Selector2/1
  Bus Selector2/1 -> Gain/1  "<Alt meas (m)>"
  Divide/1 -> Mux/4
  Bus Selector2/3 -> Divide1/2, Divide1/1, Mux/5  "<AoA meas (rad)>"
  Divide1/1 -> Mux/6
  Bus Selector2/4 -> Mux/7  "<SS meas (rad)>"
  Gain/1 -> Mux/2
  Bus Selector2/5 -> Selector/1  "<omega_b meas (rad/s)>"
  Selector/1 -> Mux/8
  Roll Multilayer NN/1(v_ad_comp) -> v_ad_comp/1
  "   "/1 -> Roll Multilayer NN/8(Theta_2)
  B/1 -> Roll Multilayer NN/4(B)
  [P] -> Roll Multilayer NN/3(P)
  v_ad^ prev/1 -> Mux/12
  Roll Multilayer NN/4(Theta_1_update) -> To Workspace/1, Memory2/1
  Roll Multilayer NN/2(v_ad) -> Terminator/1
  Divide2/1 -> [P]
  Bus Selector1/4 -> Divide2/2  "<K_b_p>"
  Constant2/1 -> Divide2/1
  Bus Selector2/2 -> Divide/2, Divide/1, Mux/3  "<Mach>"
  Roll Multilayer NN/6(Theta_3_update) -> "  "/1, " "/1
  "  "/1 -> Roll Multilayer NN/9(Theta_3)
  Roll Multilayer NN/5(Theta_2_update) -> To Workspace1/1, "   "/1
  Memory2/1 -> Roll Multilayer NN/7(Theta_1)
  Roll_learning rate/1 -> Roll Multilayer NN/5(Roll_learnign_rate)
  Roll reg param/1 -> Roll Multilayer NN/6(Roll_reg_param)
  Mux/1 -> Display/1, Scope/1, Roll Multilayer NN/1(X_bar)
  Roll Multilayer NN/3(Z_norm_unit) -> Terminator1/1
  dem-less/1 -> Mux/11

== system F16ASYM_Controlled/Primary Controller/P controller + adaptive Isolated NN/On-line (adaptive) multi-layer NNs/Yaw Chanel/Yaw HL NN ==
  note: Be careful with dimensions of inputs!!!
      | NORMALIZATION!!!
  v_ad^ prev : Inport
  Yaw_chanel vars : Inport  Port=2
  All_meas : Inport  Port=3
  Yaw_learning rate : Inport  Port=4
  Yaw reg param : Inport  Port=5
  Bus Selector1 : BusSelector  OutputSignals=beta_chanel vars.beta_err,r_chanel vars.r_err,beta_chanel vars.beta_sf,beta_chanel vars.beta_sf_dot,r_chanel vars.r_sf_dot,beta_chanel vars.K_b_beta,r_chanel vars.K_b_r
  Bus Selector2 : BusSelector  OutputSignals=signal1.Alt meas (m),signal2.Mach,signal1.AoA meas (rad),signal1.Euler meas (rad)
  Constant : Constant
  Constant1 : Constant  Value=[0;1]
  Display : Display
  Divide : Product  Inputs=**
  Gain : Gain  Gain=1/15000
  Memory2 : Memory  X0=V_yaw_last
  Memory3 : Memory  X0=W_yaw_last
  Mux : Mux  Inputs=12
  Mux1 : Mux  Inputs=2
  Mux2 : Mux  Inputs=2
  Scope : Scope
      settings: YMin=-0.25  YMax=3.75  SaveName=ScopeData17
  Selector : Selector  InputPortWidth=3
  Terminator : Terminator
  Terminator1 : Terminator
  To Workspace : ToWorkspace  VariableName=V_yaw_last  SampleTime=-1
      settings: MaxDataPoints=1
  To Workspace1 : ToWorkspace  VariableName=W_yaw_last  SampleTime=-1
      settings: MaxDataPoints=1
  Yaw NN : MATLAB Function  TreatAsAtomicUnit=on
  dem-less1 : Gain  Gain=T_sim
  dem-less2 : Gain  Gain=T_sim^2
  v_ad_comp : Outport
  wires:
  Mux2/1 -> [Ks]
  Bus Selector1/6 -> Mux2/1  "<K_b_beta>"
  Bus Selector1/7 -> Mux2/2  "<K_b_r>"
  Mux1/1 -> Yaw NN/2(e)  "e"
  Divide/1 -> Mux/4
  Bus Selector2/1 -> Gain/1  "<Alt meas (m)>"
  All_meas/1 -> Bus Selector2/1
  Constant/1 -> Mux/1
  Yaw reg param/1 -> Yaw NN/6(Long_reg_param)
  Yaw_learning rate/1 -> Yaw NN/5(Long_learnign_rate)
  Yaw_chanel vars/1 -> Bus Selector1/1
  Yaw NN/1(v_ad_comp) -> v_ad_comp/1
  Yaw NN/4(W_update) -> Memory3/1, To Workspace1/1
  Memory2/1 -> Yaw NN/8(V)
  Memory3/1 -> Yaw NN/7(W)
  Constant1/1 -> Yaw NN/4(B)
  [Ks] -> Yaw NN/3(Ks)
  v_ad^ prev/1 -> Mux/12
  Yaw NN/5(V_update) -> Memory2/1, To Workspace/1
  Yaw NN/2(v_ad) -> Terminator/1
  Bus Selector2/4 -> Selector/1  "<Euler meas (rad)>"
  Gain/1 -> Mux/2
  Bus Selector2/2 -> Divide/2, Divide/1, Mux/3  "<Mach>"
  Bus Selector2/3 -> Mux/5  "<AoA meas (rad)>"
  Selector/1 -> Mux/6
  Bus Selector1/5 -> dem-less2/1  "<r_sf_dot>"
  Bus Selector1/2 -> Mux1/2, Mux/8  "<r_err>"
  Bus Selector1/4 -> dem-less1/1  "<beta_sf_dot>"
  Bus Selector1/1 -> Mux1/1, Mux/7  "<beta_err>"
  Bus Selector1/3 -> Mux/9  "<beta_sf>"
  Mux/1 -> Display/1, Scope/1, Yaw NN/1(X_bar)
  Yaw NN/3(Z_norm_unit) -> Terminator1/1
  dem-less1/1 -> Mux/10
  dem-less2/1 -> Mux/11

== system F16ASYM_Controlled/Primary Controller/P controller + adaptive Isolated NN/On-line (adaptive) multi-layer NNs SIMPL/Long Chanel/Long HL NN A_w_z ==
  note: Be careful with dimensions of inputs!!!
      | NORMALIZATION!!!
  v_ad^ prev : Inport
  Long_chanel vars : Inport  Port=2
  All_meas : Inport  Port=3
  Long_learning rate : Inport  Port=4
  Long reg param : Inport  Port=5
  Bus Selector1 : BusSelector  OutputSignals=A_chanel vars.A_err,q_chanel_vars.q_err,A_chanel vars.A_sf,A_chanel vars.A_sf_dot,q_chanel_vars.q_sf_dot,A_chanel vars.K_b_A,q_chanel_vars.K_b_q,A_chanel vars.FactorF
  Bus Selector2 : BusSelector  OutputSignals=signal1.Alt meas (m),signal2.Mach
  Constant : Constant
  Constant1 : Constant  Value=[0;1]
  Divide : Product  Inputs=**
  Long NN : MATLAB Function  TreatAsAtomicUnit=on
  Memory2 : Memory  X0=V_long_lastA_w_z
  Memory3 : Memory  X0=W_long_lastA_w_z
  Mux : Mux  Inputs=10
  Mux1 : Mux  Inputs=2
  Mux2 : Mux  Inputs=2
  Scope : Scope
      settings: YMin=0  YMax=0.003  SaveName=ScopeData13
  Terminator : Terminator
  Terminator1 : Terminator
  To Workspace : ToWorkspace  VariableName=V_long_lastA_w_z  SampleTime=-1
      settings: MaxDataPoints=1
  To Workspace1 : ToWorkspace  VariableName=W_long_lastA_w_z  SampleTime=-1
      settings: MaxDataPoints=1
  dim-less : Gain  Gain=T_sim
  dim-less1 : Gain  Gain=T_sim^2
  scaling : Gain  Gain=1/15000
  scaling1 : Gain  Gain=1/(9*9.81)
  scaling2 : Gain  Gain=1/(9*9.81)
  scaling3 : Gain  Gain=1/(9*9.81)
  v_ad_comp : Outport
  wires:
  dim-less1/1 -> Mux/9
  dim-less/1 -> scaling3/1
  Long NN/3(Z_norm_unit) -> Terminator1/1
  scaling3/1 -> Mux/8
  scaling1/1 -> Mux/7
  scaling2/1 -> Mux/5
  Bus Selector1/8 -> Long NN/3(F)  "<FactorF>"
  Mux2/1 -> [Ks]
  Bus Selector1/6 -> Mux2/1  "<K_b_A>"
  Bus Selector1/7 -> Mux2/2  "<K_b_q>"
  Mux1/1 -> Long NN/2(e)  "e"
  Bus Selector1/5 -> dim-less1/1  "<q_sf_dot>"
  Bus Selector1/4 -> dim-less/1  "<A_sf_dot>"
  Bus Selector1/3 -> scaling1/1  "<A_sf>"
  Bus Selector1/2 -> Mux/6, Mux1/2  "<q_err>"
  Bus Selector1/1 -> scaling2/1, Mux1/1  "<A_err>"
  Bus Selector2/2 -> Divide/1, Divide/2, Mux/3  "<Mach>"
  scaling/1 -> Mux/2
  Divide/1 -> Mux/4
  Bus Selector2/1 -> scaling/1  "<Alt meas (m)>"
  All_meas/1 -> Bus Selector2/1
  Constant/1 -> Mux/1
  Long reg param/1 -> Long NN/7(Long_reg_param)
  Long_learning rate/1 -> Long NN/6(Long_learnign_rate)
  Long_chanel vars/1 -> Bus Selector1/1
  Mux/1 -> Long NN/1(X_bar), Scope/1
  Long NN/1(v_ad_comp) -> v_ad_comp/1
  Long NN/4(W_update) -> Memory3/1, To Workspace1/1
  Memory2/1 -> Long NN/9(V)
  Memory3/1 -> Long NN/8(W)
  Constant1/1 -> Long NN/5(B)
  [Ks] -> Long NN/4(Ks)
  v_ad^ prev/1 -> Mux/10
  Long NN/5(V_update) -> Memory2/1, To Workspace/1
  Long NN/2(v_ad) -> Terminator/1

== system F16ASYM_Controlled/Primary Controller/P controller + adaptive Isolated NN/On-line (adaptive) multi-layer NNs SIMPL/Long Chanel/Long HL NN AoA ==
  note: Be careful with dimensions of inputs!!!
      | NORMALIZATION!!!
  v_ad^ prev : Inport
  Long_chanel vars : Inport  Port=2
  All_meas : Inport  Port=3
  Long_learning rate : Inport  Port=4
  Long reg param : Inport  Port=5
  Bus Selector1 : BusSelector  OutputSignals=alpha_chanel vars.alpha_err,q_chanel_vars.q_err,alpha_chanel vars.alpha_sf,alpha_chanel vars.alpha_sf_dot,q_chanel_vars.q_sf_dot,alpha_chanel vars.K_b_alpha,q_chanel_vars.K_b_q
  Bus Selector2 : BusSelector  OutputSignals=signal1.Alt meas (m),signal2.Mach
  Constant : Constant
  Constant1 : Constant  Value=[0;1]
  Display : Display
  Divide : Product  Inputs=**
  Gain : Gain  Gain=1/15000
  Long NN : MATLAB Function  TreatAsAtomicUnit=on
  Memory2 : Memory  X0=V_long_lastAoA
  Memory3 : Memory  X0=W_long_lastAoA
  Mux : Mux  Inputs=10
  Mux1 : Mux  Inputs=2
  Mux2 : Mux  Inputs=2
  Scope : Scope
      settings: YMin=-0.7  YMax=1  SaveName=ScopeData18
  Terminator : Terminator
  Terminator1 : Terminator
  To Workspace : ToWorkspace  VariableName=V_long_lastAoA  SampleTime=-1
      settings: MaxDataPoints=1
  To Workspace1 : ToWorkspace  VariableName=W_long_lastAoA  SampleTime=-1
      settings: MaxDataPoints=1
  v_ad_comp : Outport
  wires:
  Mux/1 -> Long NN/1(X_bar), Display/1, Scope/1
  Long NN/3(Z_norm_unit) -> Terminator1/1
  Mux2/1 -> [Ks]
  Bus Selector1/6 -> Mux2/1  "<K_b_alpha>"
  Bus Selector1/7 -> Mux2/2  "<K_b_q>"
  Mux1/1 -> Long NN/2(e)  "e"
  Bus Selector1/5 -> Mux/9  "<q_sf_dot>"
  Bus Selector1/4 -> Mux/8  "<alpha_sf_dot>"
  Bus Selector1/3 -> Mux/7  "<alpha_sf>"
  Bus Selector1/2 -> Mux/6, Mux1/2  "<q_err>"
  Bus Selector1/1 -> Mux/5, Mux1/1  "<alpha_err>"
  Bus Selector2/2 -> Divide/1, Divide/2, Mux/3  "<Mach>"
  Gain/1 -> Mux/2
  Divide/1 -> Mux/4
  Bus Selector2/1 -> Gain/1  "<Alt meas (m)>"
  All_meas/1 -> Bus Selector2/1
  Constant/1 -> Mux/1
  Long reg param/1 -> Long NN/6(Long_reg_param)
  Long_learning rate/1 -> Long NN/5(Long_learnign_rate)
  Long_chanel vars/1 -> Bus Selector1/1
  Long NN/1(v_ad_comp) -> v_ad_comp/1
  Long NN/4(W_update) -> Memory3/1, To Workspace1/1
  Memory2/1 -> Long NN/8(V)
  Memory3/1 -> Long NN/7(W)
  Constant1/1 -> Long NN/4(B)
  [Ks] -> Long NN/3(Ks)
  v_ad^ prev/1 -> Mux/10
  Long NN/5(V_update) -> Memory2/1, To Workspace/1
  Long NN/2(v_ad) -> Terminator/1

== system F16ASYM_Controlled/Primary Controller/P controller + adaptive Isolated NN/On-line (adaptive) multi-layer NNs SIMPL/Roll NN/Roll 1HL NN ==
  note: Be careful with dimensions of inputs!!!
      | NORMALIZATION!!!
  v_ad^ prev : Inport
  p_chanel vars : Inport  Port=2
  All_meas : Inport  Port=3
  Roll_learning rate : Inport  Port=4
  Roll reg param : Inport  Port=5
  Bus Selector1 : BusSelector  OutputSignals=p_err,p_sf,p_sf_dot,K_b_p
  Bus Selector2 : BusSelector  OutputSignals=signal1.AoA meas (rad),signal1.SS meas (rad),signal1.omega_b meas (rad/s)
  Constant : Constant
  Constant1 : Constant
  Constant2 : Constant
  Display : Display
  Divide2 : Product  Inputs=*/
  Memory2 : Memory  X0=V_roll_lastMOD
  Memory3 : Memory  X0=W_roll_lastMOD
  Mux : Mux  Inputs=8
  Roll NN : MATLAB Function  TreatAsAtomicUnit=on
  Scope : Scope
      settings: YMin=-0.5  YMax=6  SaveName=ScopeData15
  Selector : Selector  InputPortWidth=3  Indices=3
  Terminator : Terminator
  Terminator1 : Terminator
  To Workspace : ToWorkspace  VariableName=V_roll_lastMOD  SampleTime=-1
      settings: MaxDataPoints=1
  To Workspace1 : ToWorkspace  VariableName=W_roll_lastMOD  SampleTime=-1
      settings: MaxDataPoints=1
  dem-less : Gain  Gain=T_sim
  v_ad_comp : Outport
  wires:
  dem-less/1 -> Mux/7
  Roll NN/3(Z_norm_unit) -> Terminator1/1
  Selector/1 -> Mux/4
  Bus Selector2/3 -> Selector/1  "<omega_b meas (rad/s)>"
  Bus Selector2/2 -> Mux/3  "<SS meas (rad)>"
  Bus Selector2/1 -> Mux/2  "<AoA meas (rad)>"
  All_meas/1 -> Bus Selector2/1
  Constant/1 -> Mux/1
  Roll reg param/1 -> Roll NN/6(Roll_reg_param)
  Roll_learning rate/1 -> Roll NN/5(Roll_learnign_rate)
  p_chanel vars/1 -> Bus Selector1/1
  Bus Selector1/2 -> Mux/6  "<p_sf>"
  Bus Selector1/3 -> dem-less/1  "<p_sf_dot>"
  Bus Selector1/1 -> Mux/5, Roll NN/2(e)  "<p_err>"
  Mux/1 -> Display/1, Scope/1, Roll NN/1(X_bar)
  Roll NN/1(v_ad_comp) -> v_ad_comp/1
  Roll NN/4(W_update) -> Memory3/1, To Workspace1/1
  Memory2/1 -> Roll NN/8(V)
  Memory3/1 -> Roll NN/7(W)
  Constant1/1 -> Roll NN/4(B)
  [P] -> Roll NN/3(P)
  v_ad^ prev/1 -> Mux/8
  Roll NN/5(V_update) -> Memory2/1, To Workspace/1
  Roll NN/2(v_ad) -> Terminator/1
  Divide2/1 -> [P]
  Bus Selector1/4 -> Divide2/2  "<K_b_p>"
  Constant2/1 -> Divide2/1
